simulink model "DCtoDC"  (R2019b)
settings: Solver=VariableStepAuto  StartTime=0.0  StopTime=6  RelTol=1e-3
model workspace (MAT data in the model file):
  Cripple1 = 0.1
  indripple = Simulink.Parameter
  indripple.Value = 0.001
  indripple.DataType = 'auto'
  indripple.DocUnits = 'H'
  indripple.Dimensions = [1 1]
undefined symbols (not defined in the file): sigbuilder_block
libraries: powerlib x22, powerlib_meascontrol x1
settings Model: OrderedModelArguments=off  Creator=Nicholas  LastModifiedBy=Nicholas
settings SolverCC: ZeroCrossAlgorithm=Adaptive
settings DataIOCC: ReturnWorkspaceOutputs=off
settings DebuggingCC: IgnoredZcDiagnostic=none

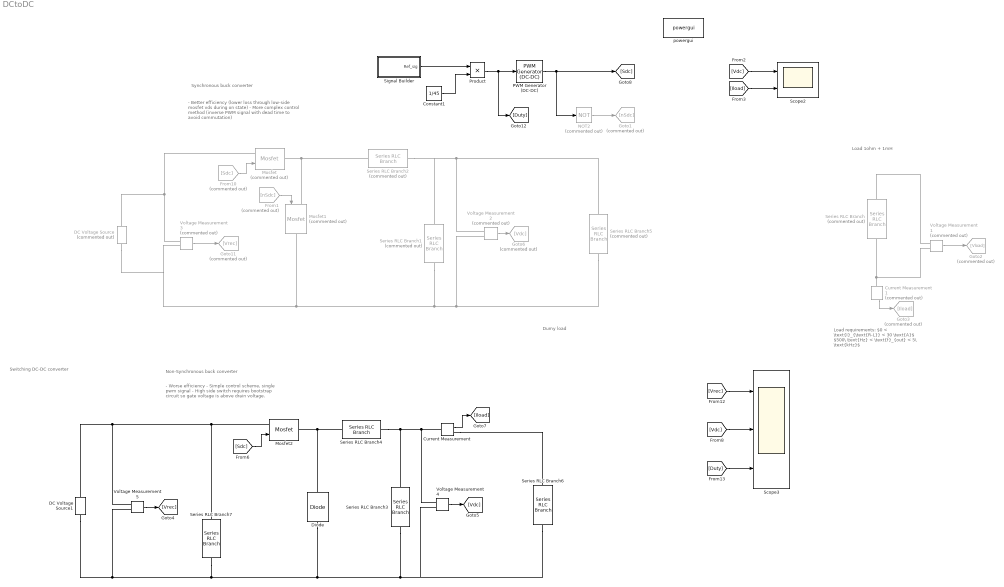
== system DCtoDC ==
  note: Load
      | 1ohm + 1mH
  note: Load requirements:
      | $0 < \text{I}_{\text{R-L}} < 30 \text{A}$
      | $500\ \text{Hz} < \text{f}_{out} < 5\ \text{kHz}$
  note: Switching DC-DC converter
  note: - Better efficiency (lower loss through low-side mosfet vds during on state)
      | - More complex control method (inverse PWM signal with dead time to avoid commutation)
  note: Dumy load
  note: Synchronous buck converter
  note: Non-Synchronous buck converter
  note: - Worse efficiency
      | - Simple control scheme, single pwm signal
      | - High side switch requires bootstrap circuit so gate voltage is above drain voltage.
  Constant1 : Constant  Value=1/45
  Current Measurement : powerlib/Measurements/Current Measurement  PhasorSimulation=off  OutputType=Complex  PSBequivalent=0
      settings: SourceProductName=Simscape Electrical
  Current Measurement1 : powerlib/Measurements/Current Measurement  Commented=on  PhasorSimulation=off  OutputType=Complex  PSBequivalent=0
      settings: SourceProductName=Simscape Electrical
  DC Voltage Source : powerlib/Electrical Sources/DC Voltage Source  Commented=on  Amplitude=50  Measurements=None
      settings: SourceProductName=Simscape Electrical
  DC Voltage Source1 : powerlib/Electrical Sources/DC Voltage Source  Amplitude=45  Measurements=None
      settings: SourceProductName=Simscape Electrical
  Diode : powerlib/Power Electronics/Diode  Ron=0.019  Lon=0  Vf=0.55  IC=0  UseSnubber=0  Rs=5000  Cs=250e-9  Measurements=off
      settings: SourceProductName=Simscape Electrical
  From1 : From  Commented=on  GotoTag=nSdc
  From10 : From  Commented=on  GotoTag=Sdc
  Goto1 : Goto  Commented=on  GotoTag=nSdc
  Goto11 : Goto  Commented=on  GotoTag=Vrec
  Goto2 : Goto  Commented=on  GotoTag=Vload
  Goto3 : Goto  Commented=on  GotoTag=Iload
  Goto6 : Goto  Commented=on  GotoTag=Vdc
  Mosfet : powerlib/Power Electronics/Mosfet  Commented=on  Ron=0.1  Lon=0  Rd=0.01  Vfd=0  IC=0  Rs=1e5  Cs=inf  Measurements=off
      settings: SourceProductName=Simscape Electrical
  Mosfet1 : powerlib/Power Electronics/Mosfet  Commented=on  Ron=0.1  Lon=0  Rd=0.01  Vfd=0  IC=0  Rs=1e5  Cs=inf  Measurements=off
      settings: SourceProductName=Simscape Electrical
  Mosfet2 : powerlib/Power Electronics/Mosfet  Ron=0.002  Lon=0  Rd=0.01  Vfd=1.3  IC=0  Rs=1e5  Cs=inf  Measurements=off
      settings: SourceProductName=Simscape Electrical
  NOT2 : Logic  Commented=on  Operator=NOT  IconShape=distinctive  AllPortsSameDT=off  OutDataTypeStr=boolean
  PWM Generator (DC-DC) : powerlib_meascontrol/Pulse & Signal Generators/PWM Generator (DC-DC)  Fsw=270000  Ts=0
      settings: SourceProductName=Simscape Electrical
  Product : Product
  Scope2 : Scope  NumInputPorts=2
  Scope3 : Scope  NumInputPorts=3
  Series RLC Branch : powerlib/Elements/Series RLC Branch  Commented=on  LConnTagsString=__new0  RConnTagsString=__new0  BranchType=RL  Resistance=1  Inductance=0.1e-3  SetiL0=off  InitialCurrent=0  Capacitance=1e-6  Setx0=off  InitialVoltage=0  Measurements=None
      settings: SourceProductName=Simscape Electrical
  Series RLC Branch1 : powerlib/Elements/Series RLC Branch  Commented=on  LConnTagsString=__new0  RConnTagsString=__new0  BranchType=C  Resistance=1  Inductance=0.1e-3  SetiL0=off  InitialCurrent=0  Capacitance=0.002  Setx0=off  InitialVoltage=0  Measurements=None
      settings: SourceProductName=Simscape Electrical
  Series RLC Branch2 : powerlib/Elements/Series RLC Branch  Commented=on  LConnTagsString=__new0  RConnTagsString=__new0  BranchType=L  Resistance=1  Inductance=0.1e-3  SetiL0=off  InitialCurrent=0  Capacitance=0.002  Setx0=off  InitialVoltage=0  Measurements=None
      settings: SourceProductName=Simscape Electrical
  Series RLC Branch3 : powerlib/Elements/Series RLC Branch  LConnTagsString=__new0  RConnTagsString=__new0  BranchType=C  Resistance=1  Inductance=0.1e-3  SetiL0=off  InitialCurrent=0  Capacitance=470e-9  Setx0=off  InitialVoltage=0  Measurements=None
      settings: SourceProductName=Simscape Electrical
  Series RLC Branch4 : powerlib/Elements/Series RLC Branch  LConnTagsString=__new0  RConnTagsString=__new0  BranchType=RL  Resistance=0.00088  Inductance=6.8e-6  SetiL0=off  InitialCurrent=0  Capacitance=0.002  Setx0=off  InitialVoltage=0  Measurements=None
      settings: SourceProductName=Simscape Electrical
  Series RLC Branch5 : powerlib/Elements/Series RLC Branch  Commented=on  LConnTagsString=__new0  RConnTagsString=__new0  BranchType=RL  Resistance=1  Inductance=0.1e-3  SetiL0=off  InitialCurrent=0  Capacitance=0.002  Setx0=off  InitialVoltage=0  Measurements=None
      settings: SourceProductName=Simscape Electrical
  Series RLC Branch6 : powerlib/Elements/Series RLC Branch  LConnTagsString=__new0  RConnTagsString=__new0  BranchType=RL  Resistance=1  Inductance=0.1e-3  SetiL0=off  InitialCurrent=0  Capacitance=0.002  Setx0=off  InitialVoltage=0  Measurements=None
      settings: SourceProductName=Simscape Electrical
  Series RLC Branch7 : powerlib/Elements/Series RLC Branch  LConnTagsString=__new0  RConnTagsString=__new0  BranchType=RC  Resistance=0.12  Inductance=0.1e-3  SetiL0=off  InitialCurrent=0  Capacitance=1.87e-6  Setx0=off  InitialVoltage=0  Measurements=None
      settings: SourceProductName=Simscape Electrical
  Signal Builder : Subsystem  Tag=STV Subsys  LoadFcn=sigbuilder_block('load');  StartFcn=sigbuilder_block('start');  StopFcn=sigbuilder_block('stop');  ClipboardFcn=sigbuilder_block('clipboard');  mask(Sigbuilder block){tuvar=[0:10]}
      mask help: Simulink:masks:SigbuilderBlock_MD
      mask init:
      | if ~strcmp(get_param(bdroot(gcbh),'SimulationStatus'),'stopped') tuvar = sigbuilder_block('maskInit'); end
      settings: CopyFcn=sigbuilder_block('copy');  DeleteFcn=sigbuilder_block('delete');  ModelCloseFcn=sigbuilder_block('modelClose');  PreSaveFcn=sigbuilder_block('preSave');  PauseFcn=sigbuilder_block('pause');  ContinueFcn=sigbuilder_block('continue');  NameChangeFcn=sigbuilder_block('namechange');  OpenFcn=sigbuilder_block('open',[581.25 327.75 550.5 318.75 ]);  CloseFcn=sigbuilder_block('close');
      mask Display: plot(0, 0, 100, 100,[2, 2, 32, 32, 2], [68, 8, 8, 68, 68],[32, 2], [38, 38], [32, 19, 2],[53, 60, 44], [32, 17, 17, 2],[16, 16, 31, 31]);txt = getActiveGroup(gcbh);text(2, 100, txt,'verticalAlignment', 'top');
  Voltage Measurement1 : powerlib/Measurements/Voltage Measurement  Commented=on  PhasorSimulation=off  OutputType=Complex  PSBequivalent=0
      settings: SourceProductName=Simscape Electrical
  Voltage Measurement2 : powerlib/Measurements/Voltage Measurement  Commented=on  PhasorSimulation=off  OutputType=Complex  PSBequivalent=0
      settings: SourceProductName=Simscape Electrical
  Voltage Measurement3 : powerlib/Measurements/Voltage Measurement  Commented=on  PhasorSimulation=off  OutputType=Complex  PSBequivalent=0
      settings: SourceProductName=Simscape Electrical
  Voltage Measurement4 : powerlib/Measurements/Voltage Measurement  PhasorSimulation=off  OutputType=Complex  PSBequivalent=0
      settings: SourceProductName=Simscape Electrical
  Voltage Measurement5 : powerlib/Measurements/Voltage Measurement  PhasorSimulation=off  OutputType=Complex  PSBequivalent=0
      settings: SourceProductName=Simscape Electrical
  powergui : powerlib/powergui  Priority=1  SimulationMode=Continuous  SampleTime=50e-6  frequency=60  Iterations=50  frequencyindice=0  Pbase=100e6  ErrMax=1e-4  UnitsV=kV  UnitsW=MW  buscounter=0  FunctionMessages=off  echomessages=off  EnableUseOfTLC=off  CurrentSourceSwitches=off  DisableSnubberDevices=off  DisableRonSwitches=off  DisableVfSwitches=off  DisplayEquations=off  AutomaticDiscreteSolvers=off  SolverType=Tustin/Backward Euler (TBE)  Interpol=off  ExternalGateDelay=off  methode=off  Ts=100  x0status=blocks  SPID=on  SwTol=0  HookPort=off  NonlinearTolerance=1e-4  nMaxIteration=100  ContinueOnMaxIteration=off  RestoreLinks=warning  ResistiveCurrentMeasurement=off  Frange=[0:2:500]  Ylog=off  Xlog=on  ShowGrid=off  save=off  variable=ZData  structure=ScopeData  ZoomFFT=on  StartTime=0.0  cycles=1  DisplayStyle=1  fundamental=50  FreqAxis=off  MaxFrequency=1000  frequencyindicesteady=1  RmsSteady=1  display=off
      settings: SourceProductName=Simscape Electrical
  wires:
  Voltage Measurement1/1 -> Goto2/1
  Current Measurement1/1 -> Goto3/1
  Voltage Measurement2/1 -> Goto6/1
  PWM Generator (DC-DC)/1 -> [Sdc], NOT2/1
  Signal Builder/1(Ref_sig) -> Product/1
  Constant1/1 -> Product/2
  Product/1 -> [Duty], PWM Generator (DC-DC)/1
  [Vdc] -> Scope2/1
  [Iload] -> Scope2/2
  From10/1 -> Mosfet/1
  From1/1 -> Mosfet1/1
  [Vdc] -> Scope3/2
  Voltage Measurement3/1 -> Goto11/1
  [Vrec] -> Scope3/1
  [Duty] -> Scope3/3
  Voltage Measurement4/1 -> [Vdc]
  Voltage Measurement5/1 -> [Vrec]
  [Sdc] -> Mosfet2/1
  Current Measurement/1 -> [Iload]
  NOT2/1 -> Goto1/1
  connections:
  Current Measurement1/LConn1 -- Voltage Measurement1/LConn2 -- Series RLC Branch/RConn1
  Series RLC Branch5/RConn1 -- Voltage Measurement2/LConn2 -- Series RLC Branch1/RConn1 -- DC Voltage Source/LConn1 -- Voltage Measurement3/LConn2 -- Mosfet1/RConn1
  Series RLC Branch5/LConn1 -- Voltage Measurement2/LConn1 -- Series RLC Branch1/LConn1 -- Series RLC Branch2/RConn1
  Voltage Measurement1/LConn1 -- Series RLC Branch/LConn1
  Series RLC Branch2/LConn1 -- Mosfet/RConn1 -- Mosfet1/LConn1
  Voltage Measurement3/LConn1 -- DC Voltage Source/RConn1 -- Mosfet/LConn1
  Voltage Measurement5/LConn2 -- DC Voltage Source1/LConn1 -- Series RLC Branch7/RConn1 -- Diode/LConn1 -- Series RLC Branch6/RConn1 -- Voltage Measurement4/LConn2 -- Series RLC Branch3/RConn1
  Series RLC Branch3/LConn1 -- Current Measurement/LConn1 -- Voltage Measurement4/LConn1 -- Series RLC Branch4/RConn1
  Series RLC Branch4/LConn1 -- Diode/RConn1 -- Mosfet2/RConn1
  Voltage Measurement5/LConn1 -- DC Voltage Source1/RConn1 -- Series RLC Branch7/LConn1 -- Mosfet2/LConn1
  Current Measurement/RConn1 -- Series RLC Branch6/LConn1

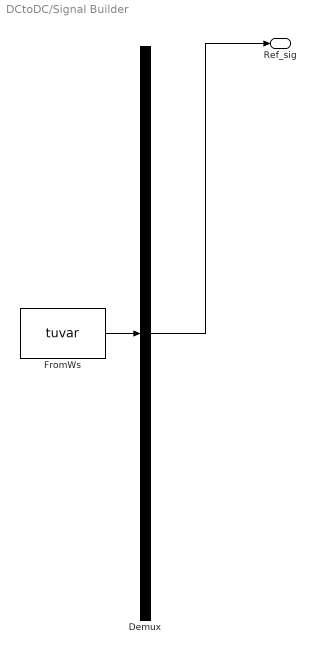
== system DCtoDC/Signal Builder ==
  Demux : Demux  Tag=STV Demux  Outputs=1
  FromWs : FromWorkspace  Tag=STV FromWs  VariableName=tuvar  SampleTime=0
      SigBuilderData=|
      | common.afterFinalStr = 'Extrapolate'
      | common.sampleTime = 0
      | dataSet.timeRange = [0 10]
      | dataSet.name = 'Group 1'
      | sbobj.Groups.Name = 'Group 1'
      | sbobj.Groups.Signals.Name = 'Ref_sig'
      | sbobj.Groups.Signals.XData = [0 1 1 3 3 5 5.5 6 6 10]
      | sbobj.Groups.Signals.YData = [3 3 20 20 10 10 18 18 0 0]
  Ref_sig : Outport  Tag=STV Outport
  wires:
  Demux/1 -> Ref_sig/1
  FromWs/1 -> Demux/1
